simulink model "Lab3Part1Model"  (R2016a)
settings: Solver=VariableStepAuto  StartTime=0.0  StopTime=10e-3  RelTol=1e-3
libraries: elec_lib x8, SimscapeMacros x5, dspstat3 x2, fl_lib x1, nesl_utility x1
settings Model: Creator=Peter  LastModifiedBy=Peter

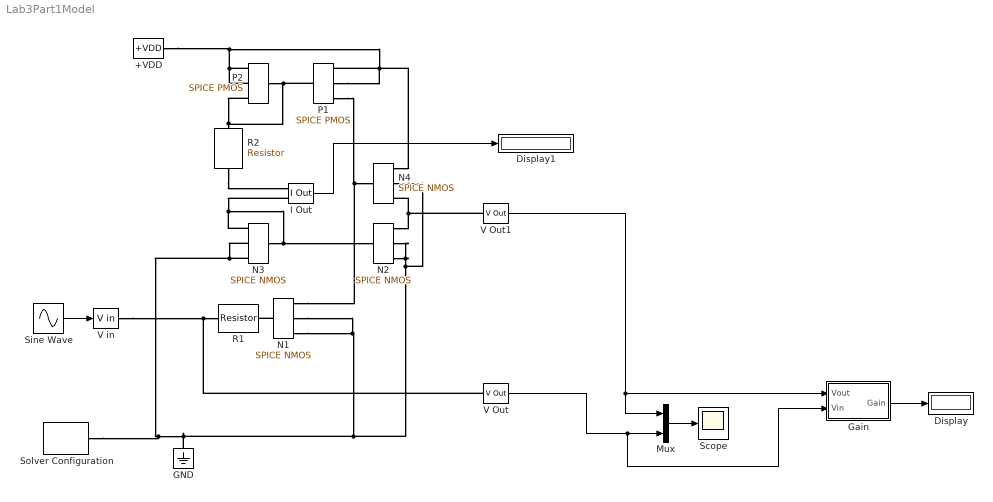
== system Lab3Part1Model ==
  +VDD : SimscapeMacros/+VDD
  Display : Display
  Display1 : Display
  GND : fl_lib/Electrical/Electrical Elements/Electrical Reference
  Gain : Subsystem
  I Out : SimscapeMacros/I Out
  Mux : Mux  Inputs=2
  N{1..4} (4 alike) : elec_lib/Additional Components/SPICE-Compatible Components/Semiconductor Devices/SPICE NMOS  AREA=1  SCALE=1  LENGTH=7.8e-6 m  WIDTH=0.138e-3 m  AD=0.161e-8 m^2  AS=0.603e-8 m^2  PD=0 m  PS=0.478e-3 m  NRD=0.3  NRS=1  LEVEL=1  VTO=0.750 V  KP=NaN A/V^2  GAMMA=1.03 V^0.50000  PHI=0.70 V  LAMBDA=0.018 1/V  RD=NaN Ohm  RS=NaN Ohm  C_param=1  CBD=1e-18 F  CBS=1e-18 F  IS=1.206e-13 A  ND=1  PB=0.9 V  CGSO=0.94e-9 F/m  CGDO=0.59e-9 F/m  CGBO=0.138e-9 F/m  RSH=10 Ohm  CJ=0.39e-3 F/m^2  MJ=0.5  CJSW=264e-12 F/m  MJSW=0.18  JS=20e-6 A/m^2  TOX=0.055e-6 m  LD=1.6e-6 m  U0=650 cm^2/s/V  FC=0.5  NSUB=1e16 1/cm^3  TPG=1  NSS=0.7e11 1/cm^2  UEXP=0  UCRIT=1e+4 V/cm  NEFF=1  DELTA=0  VMAX=1.6e5 m/s  XJ=2.0e-6 m  NFS=1.17e11 1/cm^2  ETA=0  THETA=0 1/V  KAPPA=0.2  T_param=1  TOFFSET=0 K  TFIXED=300.15 K  TMEAS=300.15 K  IC_given=1  ICVDS=0 V  ICVGS=0 V  ICVBS=0 V  MTYPE=1
  P1 : elec_lib/Additional Components/SPICE-Compatible Components/Semiconductor Devices/SPICE PMOS  AREA=1  SCALE=1  LENGTH=7.8e-6 m  WIDTH=0.138e-3 m  AD=0.161e-8 m^2  AS=0.603e-8 m^2  PD=0 m  PS=0.478e-3 m  NRD=0.3  NRS=1  LEVEL=1  VTO=-0.74 V  KP=NaN A/V^2  GAMMA=0.58 V^0.50000  PHI=0.70 V  LAMBDA=.026 1/V  RD=NaN Ohm  RS=NaN Ohm  C_param=1  CBD=1e-18 F  CBS=1e-18 F  IS=1.206e-13 A  ND=1  PB=0.90 V  CGSO=0.31e-9 F/m  CGDO=0.39e-9 F/m  CGBO=0.138e-9 F/m  RSH=90 Ohm  CJ=0.18e-3 F/m^2  MJ=0.57  CJSW=322e-12 F/m  MJSW=0.33  JS=20e-6 A/m^2  TOX=0.055e-6 m  LD=0.96e-6 m  U0=260 cm^2/s/V  FC=0.5  NSUB=1e16 1/cm^3  TPG=-1  NSS=1e11 1/cm^2  UEXP=0  UCRIT=1e+4 V/cm  NEFF=1  DELTA=0  VMAX=3.0e5 m/s  XJ=1.2e-6 m  NFS=1.06e11 1/cm^2  ETA=0  THETA=0 1/V  KAPPA=0.2  T_param=1  TOFFSET=0 K  TFIXED=300.15 K  TMEAS=300.15 K  IC_given=1  ICVDS=0 V  ICVGS=0 V  ICVBS=0 V  MTYPE=-1
  P2 : elec_lib/Additional Components/SPICE-Compatible Components/Semiconductor Devices/SPICE PMOS  AREA=1  SCALE=1  LENGTH=7.8e-6 m  WIDTH=0.138e-3 m  AD=0.161e-8 m^2  AS=0.603e-8 m^2  PD=0 m  PS=0.478e-3 m  NRD=0.3  NRS=1  LEVEL=1  VTO=-0.74 V  KP=NaN A/V^2  GAMMA=0.58 V^0.50000  PHI=0.70 V  LAMBDA=.026 1/V  RD=NaN Ohm  RS=NaN Ohm  C_param=1  CBD=1e-18 F  CBS=1e-18 F  IS=1.206e-13 A  ND=1  PB=0.90 V  CGSO=0.31e-9 F/m  CGDO=0.39e-9 F/m  CGBO=0.138e-9 F/m  RSH=90 Ohm  CJ=0.18e-3 F/m^2  MJ=0.57  CJSW=322e-12 F/m  MJSW=0.33  JS=20e-6 A/m^2  TOX=0.055e-6 m  LD=0.96e-6 m  U0=260 cm^2/s/V  FC=0.5  NSUB=1e16 1/cm^3  TPG=-1  NSS=1e11 1/cm^2  UEXP=0  UCRIT=1e+4 V/cm  NEFF=1  DELTA=0  VMAX=3.0e5 m/s  XJ=1.2e-6 m  NFS=1.06e11 1/cm^2  ETA=0  THETA=0 1/V  KAPPA=0.2  T_param=1  TOFFSET=0 K  TFIXED=300.15 K  TMEAS=300.15 K  IC_given=1  ICVDS=0 V  ICVGS=0 V  ICVBS=0 V  MTYPE=-1
  R1 : elec_lib/Passive Devices/Resistor  R=10e3 Ohm  R_tol=5  enable_R_tol=0  tol_distribution=1  nSigma=4  enable_operating_limits=0  operating_limit_action=2  max_working_voltage=100 V  power_rating=1 W  enable_faults=0  fault_action=1  R_faulted=Inf Ohm  enable_temporal_fault=0  t_fault=1 s  enable_behavioral_fault=0  max_permissible_current=1 A  t_fail_on_current=1 s  noise_mode=0  sample_time=0.001 s  repeatability=1  auto_seed=1254553298  user_seed=0  Tdevice=25 degC  alpha=0.00393 1/K  Tmeas=25 degC  thermal_mass=100 J/K  initial_temperature=25 degC  power_derating_T1=70 degC  power_derating_T2=155 degC  operating_temperature_range_vec=[ -50 150 ] degC
  R2 : elec_lib/Passive Devices/Resistor  R=73e3 Ohm  R_tol=5  enable_R_tol=0  tol_distribution=1  nSigma=4  enable_operating_limits=0  operating_limit_action=2  max_working_voltage=100 V  power_rating=1 W  enable_faults=0  fault_action=1  R_faulted=Inf Ohm  enable_temporal_fault=0  t_fault=1 s  enable_behavioral_fault=0  max_permissible_current=1 A  t_fail_on_current=1 s  noise_mode=0  sample_time=0.001 s  repeatability=1  auto_seed=2547358782  user_seed=0  Tdevice=25 degC  alpha=0.00393 1/K  Tmeas=25 degC  thermal_mass=100 J/K  initial_temperature=25 degC  power_derating_T1=70 degC  power_derating_T2=155 degC  operating_temperature_range_vec=[ -50 150 ] degC
  Scope : Scope
  Sine Wave : Sin  Amplitude=5e-3  Bias=1.15  Frequency=2*pi*1e3  SampleTime=0
  Solver Configuration : nesl_utility/Solver Configuration  PhysicalDomain=network_engine_domain  SubClassName=solver  LeftPortType=input  RightPortType=generic  Accelerate=off  Tones=[]  Harmonics=[]  SimulateNoise=off  Profile=off  UseLocalSampling=off  EnableSwitchedLinearOptims=on  FrequencyDomain=off  UseCCode=off  RelTol=0.001  AbsTol=1e-06  MinStep=1e-09  ToWorkspace=off  RevertToSquareIcSolve=off  NumHomotopyIterations=100  PhasorMode=off  PhasorModeNumHarmonics=1  OverrideAbsTol=off  DoDC=off  ResidualTolerance=1e-09  UseLocalSolver=off  LocalSolverChoice=NE_BACKWARD_EULER_ADVANCER  LocalSolverSampleTime=0.001  DoFixedCost=off  MaxNonlinIter=3  MaxModeIter=2  LinearAlgebra=Sparse  DelaysMemoryBudget=1024  AutomaticFiltering=on  FilteringTimeConstant=0.001
  V Out : SimscapeMacros/V Out
  V Out1 : SimscapeMacros/V Out
  V in : SimscapeMacros/V in
  wires:
  Mux/1 -> Scope/1
  Gain/1(Gain) -> Display/1
  V Out/1 -> Gain/2(Vin), Mux/2
  V Out1/1 -> Gain/1(Vout), Mux/1
  I Out/1 -> Display1/1
  Sine Wave/1 -> V in/1
  connections:
  N1/RConn1 -- N4/RConn2 -- N2/RConn2 -- N2/RConn1 -- Solver Configuration/RConn1 -- N3/RConn2 -- N3/RConn1 -- GND/LConn1 -- N1/RConn2
  V in/RConn1 -- V Out/LConn1 -- R1/LConn1
  N1/LConn1 -- R1/RConn1
  N3/LConn1 -- N3/RConn3 -- I Out/LConn2 -- N2/LConn1
  P2/RConn3 -- P1/LConn1 -- P2/LConn1 -- R2/LConn1
  N2/RConn3 -- N4/RConn1 -- V Out1/LConn1
  P2/RConn1 -- +VDD/RConn1 -- N4/RConn3 -- P1/RConn2 -- P1/RConn1 -- P2/RConn2
  P1/RConn3 -- N1/RConn3 -- N4/LConn1
  R2/RConn1 -- I Out/LConn1

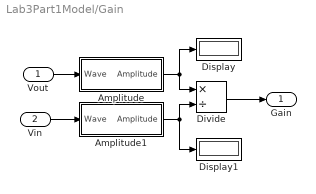
== system Lab3Part1Model/Gain ==
  Vout : Inport
  Vin : Inport  Port=2
  Amplitude : Subsystem
  Amplitude1 : Subsystem
  Display : Display
  Display1 : Display
  Divide : Product  Inputs=*/
  Gain : Outport
  wires:
  Vout/1 -> Amplitude/1(Wave)
  Divide/1 -> Gain/1
  Vin/1 -> Amplitude1/1(Wave)
  Amplitude/1(Amplitude) -> Display/1, Divide/1
  Amplitude1/1(Amplitude) -> Display1/1, Divide/2

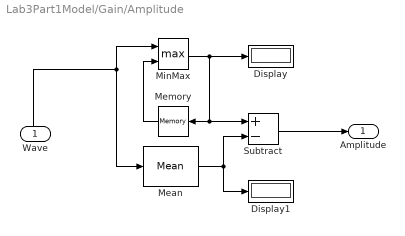
== system Lab3Part1Model/Gain/Amplitude ==
  Wave : Inport
  Display : Display
  Display1 : Display
  Mean : dspstat3/Mean  run=off  reset_popup=None  InputProcessing=Columns as channels (frame based)  directionMode=Each column  dimension=1  roiEnable=off  roiType=Rectangles  roiPortion=Entire ROI  roiOutput=Individual statistics for each ROI  roiFlag=off  outputDataTypeStr=Inherit: Same as accumulator  outputLastDataTypeStr=Inherit: Same as accumulator  outputMin=[]  outputMax=[]  roundingMode=Floor  overflowMode=off
  Memory : Memory  X0=1e-15  InheritSampleTime=on
  MinMax : MinMax  Function=max  Inputs=2
  Subtract : Sum  Inputs=+-
  Amplitude : Outport
  wires:
  Subtract/1 -> Amplitude/1
  Wave/1 -> Mean/1, MinMax/1
  Mean/1 -> Subtract/2, Display1/1
  MinMax/1 -> Display/1, Subtract/1, Memory/1
  Memory/1 -> MinMax/2

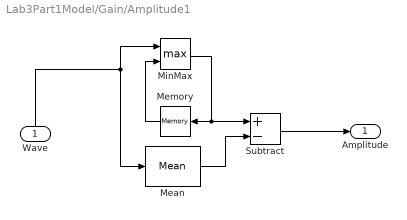
== system Lab3Part1Model/Gain/Amplitude1 ==
  Wave : Inport
  Mean : dspstat3/Mean  run=off  reset_popup=None  InputProcessing=Columns as channels (frame based)  directionMode=Each column  dimension=1  roiEnable=off  roiType=Rectangles  roiPortion=Entire ROI  roiOutput=Individual statistics for each ROI  roiFlag=off  outputDataTypeStr=Inherit: Same as accumulator  outputLastDataTypeStr=Inherit: Same as accumulator  outputMin=[]  outputMax=[]  roundingMode=Floor  overflowMode=off
  Memory : Memory  X0=1e-15  InheritSampleTime=on
  MinMax : MinMax  Function=max  Inputs=2
  Subtract : Sum  Inputs=+-
  Amplitude : Outport
  wires:
  Subtract/1 -> Amplitude/1
  Wave/1 -> Mean/1, MinMax/1
  Mean/1 -> Subtract/2
  MinMax/1 -> Subtract/1, Memory/1
  Memory/1 -> MinMax/2
